simulink model "Projekt_Marvin_Perzi_5AHEL"  (R2022b)
settings: Solver=VariableStepAuto  StartTime=0.0  StopTime=2  RelTol=1e-3
model workspace (MAT data in the model file):
  Fs = 16000
undefined symbols (not defined in the file): magnitude
libraries: dsparch4 x4, simulink x2, dspsrcs4 x2
settings Model: Creator=Josef  LastModifiedBy=Persie
settings SolverCC: AlgebraicLoopSolver=TrustRegion
settings DataIOCC: ReturnWorkspaceOutputs=off
settings DebuggingCC: UnconnectedInputMsg=warning  UnconnectedOutputMsg=warning  UnconnectedLineMsg=warning  SFMachineParentedDataDiag=warning  ArithmeticOperatorsInVariantConditions=warning
settings ModelReferenceCC: EnableRefExpFcnMdlSchedulingChecks=on
settings SFSimCC: SimUseLocalCustomCode=off  CustomCodeUndefinedFunction=UseInterfaceOnly
settings RTWCC: RTWUseLocalCustomCode=off  DLArmComputeVersion=19.05

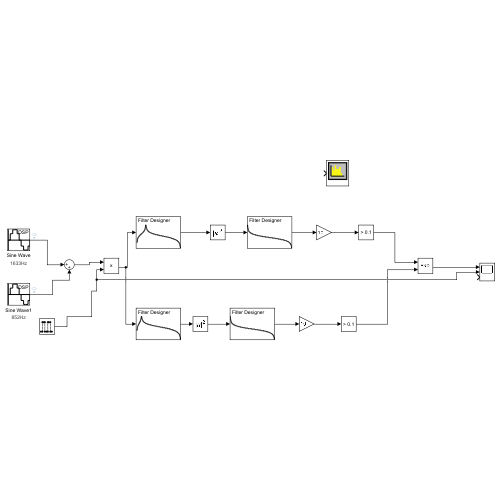
[thumbnail: Simulink's stored preview of the top-level diagram]
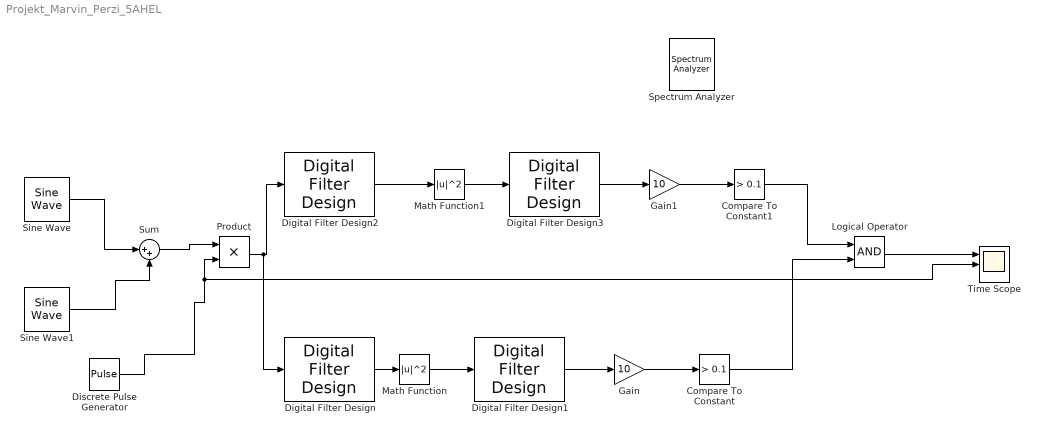
== system Projekt_Marvin_Perzi_5AHEL ==
  Compare To Constant : simulink/Logic and Bit Operations/Compare To Constant  relop=>  const=0.1  OutDataTypeStr=boolean
  Compare To Constant1 : simulink/Logic and Bit Operations/Compare To Constant  relop=>  const=0.1  OutDataTypeStr=boolean
  Digital Filter Design{,1..3} (4 alike) : dsparch4/Digital Filter Design  mwdsp_browser_bugfix_var=off
  Discrete Pulse Generator : DiscretePulseGenerator  Period=4800  PulseWidth=80  SampleTime=1/Fs
  Gain : Gain  Gain=10
  Gain1 : Gain  Gain=10
  Logical Operator : Logic  AllPortsSameDT=off  OutDataTypeStr=boolean
  Math Function : Math  Operator=magnitude^2  SignedPower=on
  Math Function1 : Math  Operator=magnitude^2  SignedPower=on
  Product : Product
  Sine Wave : dspsrcs4/Sine Wave  Amplitude=1  Frequency=1633  Phase=0  SampleMode=Discrete  OutComplex=Real  CompMethod=Trigonometric fcn  TableSize=Speed  SampleTime=1/Fs  SamplesPerFrame=1  ResetState=Restart at time zero  OutputFrames=off  dataType=double  wordLen=16  udDataType=sfix(16)  fracBitsMode=Best precision  numFracBits=15  OutDataTypeStr=double  LastOutDataTypeStr=double
      settings: AttributesFormatString=1633Hz
  Sine Wave1 : dspsrcs4/Sine Wave  Amplitude=1  Frequency=852  Phase=0  SampleMode=Discrete  OutComplex=Real  CompMethod=Trigonometric fcn  TableSize=Speed  SampleTime=1/Fs  SamplesPerFrame=1  ResetState=Restart at time zero  OutputFrames=off  dataType=double  wordLen=16  udDataType=sfix(16)  fracBitsMode=Best precision  numFracBits=15  OutDataTypeStr=double  LastOutDataTypeStr=double
      settings: AttributesFormatString=852Hz
  Spectrum Analyzer : SpectrumAnalyzer
  Sum : Sum  Inputs=|++
  Time Scope : Scope  NumInputPorts=3
  wires:
  Sine Wave/1 -> Sum/1
  Sine Wave1/1 -> Sum/2
  Digital Filter Design/1 -> Math Function/1
  Math Function/1 -> Digital Filter Design1/1
  Digital Filter Design1/1 -> Gain/1
  Gain/1 -> Compare To Constant/1
  Digital Filter Design2/1 -> Math Function1/1
  Gain1/1 -> Compare To Constant1/1
  Digital Filter Design3/1 -> Gain1/1
  Math Function1/1 -> Digital Filter Design3/1
  Discrete Pulse Generator/1 -> Time Scope/2, Product/2
  Sum/1 -> Product/1
  Product/1 -> Digital Filter Design/1, Digital Filter Design2/1
  Compare To Constant1/1 -> Logical Operator/1
  Compare To Constant/1 -> Logical Operator/2
  Logical Operator/1 -> Time Scope/1
